simulink model "System_1_2"  (R2017a)
settings: Solver=VariableStepAuto  StartTime=0.0  StopTime=1000  MaxStep=0.01  RelTol=1e-3
values from neighbouring files (symbols this model uses):
  kc = numerator(2)    [System1.m]
  kd = numerator(1)    [System1.m]
  ki = numerator(3)    [System1.m]
  r_t = b    (= 5)    [System1.m]
libraries: cstblocks x1
settings Model: Creator=dplascen  LastModifiedBy=dplascen
settings HardwareCC: ProdBitPerPointer=32  ProdBitPerSizeT=32  ProdBitPerPtrDiffT=32  ProdWordSize=32  ProdHWDeviceType=Intel->x86-32 (Windows32)

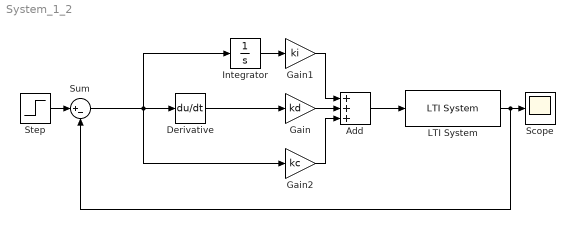
== system System_1_2 ==
  Add : Sum  Inputs=+++
  Derivative : Derivative
  Gain : Gain  Gain=kd
  Gain1 : Gain  Gain=ki
  Gain2 : Gain  Gain=kc
  Integrator : Integrator
  LTI System : cstblocks/LTI System  sys=G  IC=[]
  Scope : Scope
  Step : Step  Time=0  After=r_t  SampleTime=0
  Sum : Sum  Inputs=|+-
  wires:
  LTI System/1 -> Sum/2, Scope/1
  Step/1 -> Sum/1
  Add/1 -> LTI System/1
  Gain/1 -> Add/2
  Gain1/1 -> Add/1
  Gain2/1 -> Add/3
  Sum/1 -> Gain2/1, Integrator/1, Derivative/1
  Derivative/1 -> Gain/1
  Integrator/1 -> Gain1/1
